simulink model "MultirotorSimulation"  (R2015b)
settings: Solver=VariableStepAuto  StartTime=0.0  StopTime=100  RelTol=1e-3
undefined symbols (not defined in the file): Initial, Motor, Uav
libraries: QuaternionLibrary x7
settings Model: Creator=jban039  LastModifiedBy=jeremie
settings ModelReferenceCC: ModelReferenceMinAlgLoopOccurrences=on

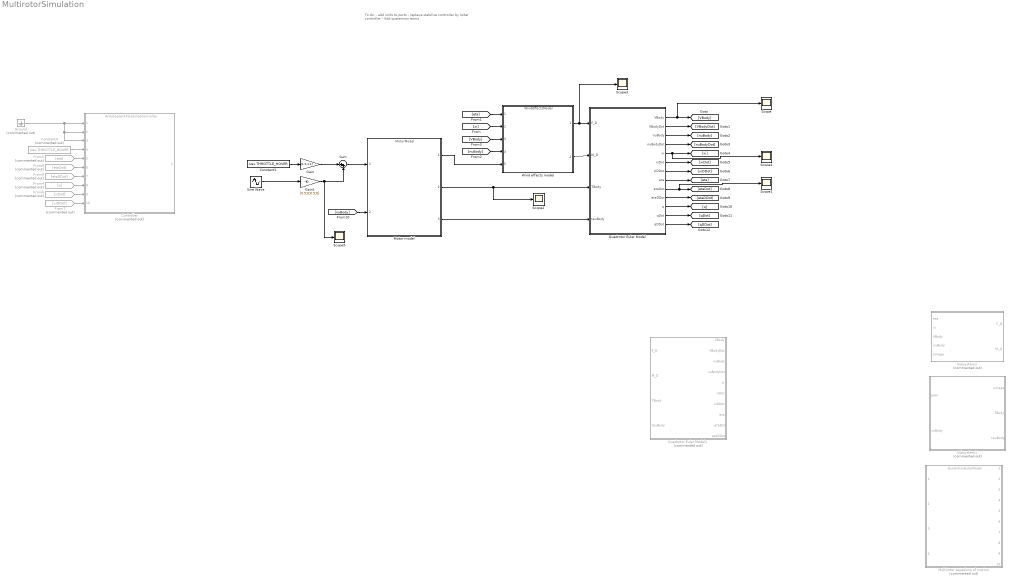
== system MultirotorSimulation ==
  note: To do:
      |
      | - add units  to ports
      | - replace stabilize controller by loiter controller
      | - Add quaternion eoms
  Constant1 : Constant  Value=Uav.THROTTLE_HOVER
  Constant4 : Constant  Commented=on  Value=Uav.THROTTLE_HOVER
  Controller : ModelReference  Commented=on  ModelNameDialog=ArduCopter33StabilizeController  SimulationMode=Normal  ModelReferenceVersion=1.9  CopyOfModelName=ArduCopter33StabilizeController
  From4 : From  Commented=on  GotoTag=xi
  From5 : From  Commented=on  GotoTag=eta
  From6 : From  Commented=on  GotoTag=xiDot
  From7 : From  Commented=on  GotoTag=xiDDot
  From8 : From  Commented=on  GotoTag=etaDot
  From9 : From  Commented=on  GotoTag=etaDDot
  Gain : Gain  Gain=[1;1;1;1]
  Gain1 : Gain  Gain=[0.5;0;0.5;0]
  Ground : Ground  Commented=on
  Motor model : ModelReference  ModelNameDialog=MotorModel  SimulationMode=Normal  ModelReferenceVersion=1.107  CopyOfModelName=MotorModel
  Multirotor equations of motion : ModelReference  Commented=on  ModelNameDialog=QuadrotorEulerModel  SimulationMode=Normal  ModelReferenceVersion=1.104  CopyOfModelName=QuadrotorEulerModel
  Quadrotor Euler Model : Subsystem
  Quadrotor Euler Model1 : Subsystem  Commented=on
  Scope{,1..5} (6 alike) : Scope
  Sine Wave : Sin  Amplitude=30  SampleTime=0
  Subsystem1 : Subsystem  Commented=on
  Subsystem2 : Subsystem  Commented=on
  Sum : Sum  Inputs=|++
  Wind effects model : ModelReference  ModelNameDialog=WindEffectsModel  SimulationMode=Normal  ModelReferenceVersion=1.49  CopyOfModelName=WindEffectsModel
  wires:
  Motor model/1 -> Wind effects model/5
  Motor model/2 -> Scope2/1, Quadrotor Euler Model/3(TBody)
  Motor model/3 -> Quadrotor Euler Model/4(tauBody)
  Wind effects model/2 -> Quadrotor Euler Model/2(M_D)
  Quadrotor Euler Model/1(VBody) -> Scope/1, [VBody]
  Quadrotor Euler Model/2(VBodyDot) -> [VBodyDot]
  Quadrotor Euler Model/3(nuBody) -> [nuBody]
  Quadrotor Euler Model/4(nuBodyDot) -> [nuBodyDot]
  Quadrotor Euler Model/5(xi) -> Scope4/1, [xi]
  Quadrotor Euler Model/6(xiDot) -> [xiDot]
  Quadrotor Euler Model/7(xiDDot) -> [xiDDot]
  Quadrotor Euler Model/8(eta) -> [eta]
  Quadrotor Euler Model/9(etaDot) -> Scope1/1, [etaDot]
  Quadrotor Euler Model/10(etaDDot) -> [etaDDot]
  [eta] -> Wind effects model/1
  [xi] -> Wind effects model/2
  [nuBody] -> Wind effects model/4
  [VBody] -> Wind effects model/3
  From5/1 -> Controller/5
  From4/1 -> Controller/8
  From6/1 -> Controller/9
  From7/1 -> Controller/10
  From8/1 -> Controller/6
  From9/1 -> Controller/7
  Ground/1 -> Controller/3, Controller/2, Controller/1
  Constant4/1 -> Controller/4
  [nuBody] -> Motor model/2
  Gain/1 -> Sum/1
  Constant1/1 -> Gain/1
  Sum/1 -> Motor model/1
  Gain1/1 -> Scope5/1, Sum/2
  Sine Wave/1 -> Gain1/1
  Quadrotor Euler Model/11(q) -> [q]
  Quadrotor Euler Model/12(qDot) -> [qDot]
  Quadrotor Euler Model/13(qDDot) -> [qDDot]
  Wind effects model/1 -> Scope3/1, Quadrotor Euler Model/1(F_D)

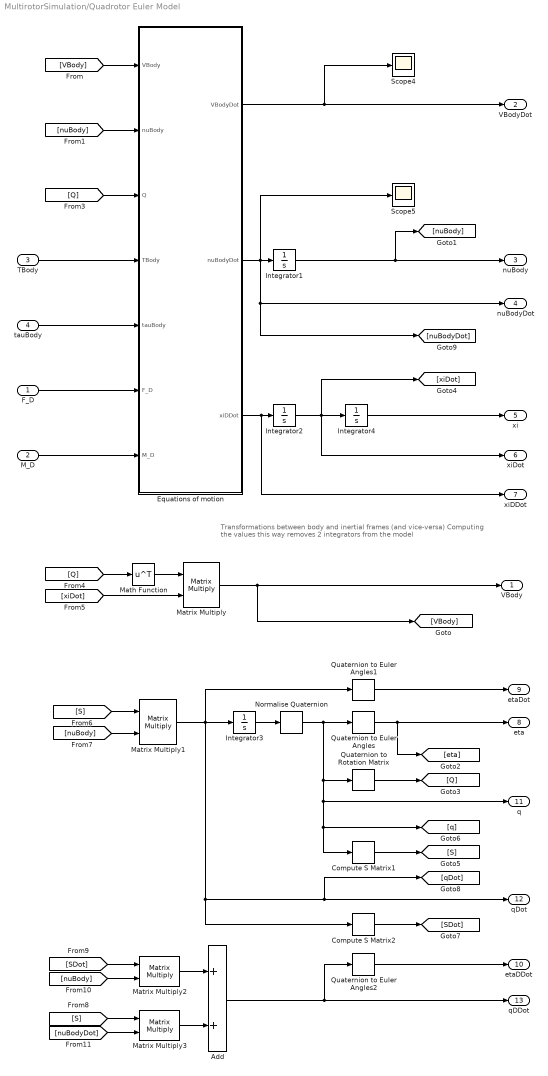
== system MultirotorSimulation/Quadrotor Euler Model ==
  note: Transformations between body and inertial frames (and vice-versa)
      | Computing the values this way removes 2 integrators from the model
  F_D : Inport
  M_D : Inport  Port=2
  TBody : Inport  Port=3
  tauBody : Inport  Port=4
  Add : Sum
  Compute S Matrix1 : QuaternionLibrary/Compute S Matrix
  Compute S Matrix2 : QuaternionLibrary/Compute S Matrix
  Equations of motion : MATLAB Function  TreatAsAtomicUnit=on
  Integrator1 : Integrator  InitialCondition=Initial.NU_BODY
  Integrator2 : Integrator  InitialCondition=Initial.XI_DOT
  Integrator3 : Integrator  InitialCondition=[0;0;0;1]
  Integrator4 : Integrator  InitialCondition=Initial.XI
  Math Function : Math  Operator=transpose  SaturateOnIntegerOverflow=on
  Matrix Multiply{,1..3} (4 alike) : Product  Multiplication=Matrix(*)
  Normalise Quaternion : QuaternionLibrary/Normalise Quaternion
  Quaternion to Euler Angles : QuaternionLibrary/Quaternion to Euler Angles
  Quaternion to Euler Angles1 : QuaternionLibrary/Quaternion to Euler Angles
  Quaternion to Euler Angles2 : QuaternionLibrary/Quaternion to Euler Angles
  Quaternion to Rotation Matrix : QuaternionLibrary/Quaternion to Rotation Matrix
  Scope4 : Scope
  Scope5 : Scope
  VBody : Outport
  VBodyDot : Outport  Port=2
  nuBody : Outport  Port=3
  nuBodyDot : Outport  Port=4
  xi : Outport  Port=5
  xiDot : Outport  Port=6
  xiDDot : Outport  Port=7
  eta : Outport  Port=8
  etaDot : Outport  Port=9
  etaDDot : Outport  Port=10
  q : Outport  Port=11
  qDot : Outport  Port=12
  qDDot : Outport  Port=13
  wires:
  Equations of motion/1(VBodyDot) -> VBodyDot/1, Scope4/1
  Integrator2/1 -> Integrator4/1, [xiDot], xiDot/1
  Integrator4/1 -> xi/1
  [nuBody] -> Equations of motion/2(nuBody)
  [VBody] -> Equations of motion/1(VBody)
  tauBody/1 -> Equations of motion/5(tauBody)
  TBody/1 -> Equations of motion/4(TBody)
  Equations of motion/3(xiDDot) -> Integrator2/1, xiDDot/1
  F_D/1 -> Equations of motion/6(F_D)
  Matrix Multiply/1 -> VBody/1, [VBody]
  M_D/1 -> Equations of motion/7(M_D)
  Integrator1/1 -> [nuBody], nuBody/1
  Equations of motion/2(nuBodyDot) -> Integrator1/1, nuBodyDot/1, [nuBodyDot], Scope5/1
  Integrator3/1 -> Normalise Quaternion/1
  Quaternion to Euler Angles/1 -> eta/1, [eta]
  Quaternion to Euler Angles1/1 -> etaDot/1
  Quaternion to Rotation Matrix/1 -> [Q]
  [Q] -> Equations of motion/3(Q)
  [Q] -> Math Function/1
  [xiDot] -> Matrix Multiply/2
  Math Function/1 -> Matrix Multiply/1
  [S] -> Matrix Multiply1/1
  [nuBody] -> Matrix Multiply1/2
  Compute S Matrix2/1 -> [SDot]
  [S] -> Matrix Multiply3/1
  Matrix Multiply1/1 -> Quaternion to Euler Angles1/1, qDot/1, [qDot], Compute S Matrix2/1, Integrator3/1
  [SDot] -> Matrix Multiply2/1
  [nuBody] -> Matrix Multiply2/2
  [nuBodyDot] -> Matrix Multiply3/2
  Matrix Multiply2/1 -> Add/1
  Matrix Multiply3/1 -> Add/2
  Add/1 -> Quaternion to Euler Angles2/1, qDDot/1
  Normalise Quaternion/1 -> Quaternion to Euler Angles/1, q/1, Compute S Matrix1/1, [q], Quaternion to Rotation Matrix/1
  Compute S Matrix1/1 -> [S]
  Quaternion to Euler Angles2/1 -> etaDDot/1

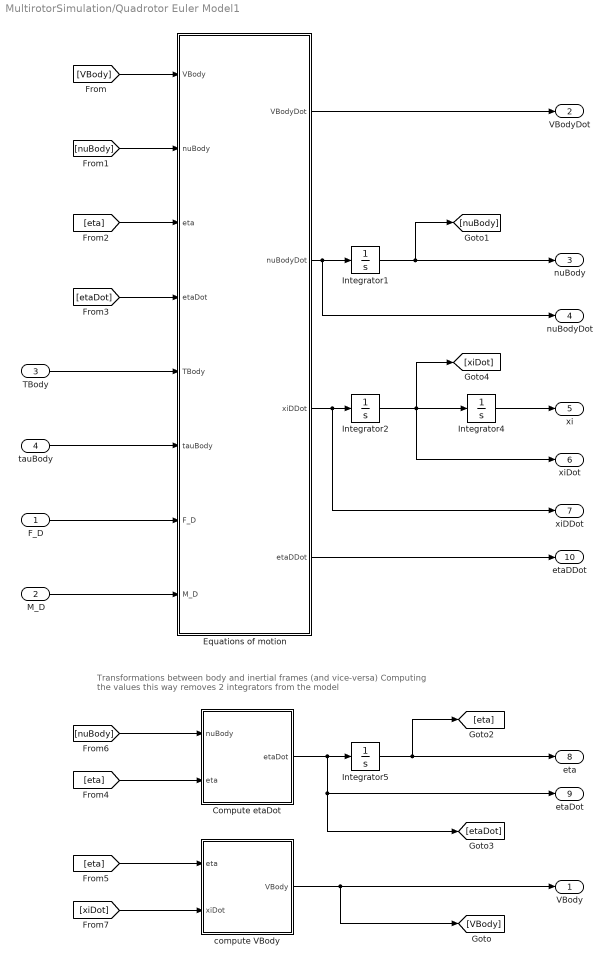
== system MultirotorSimulation/Quadrotor Euler Model1 ==
  note: Transformations between body and inertial frames (and vice-versa)
      | Computing the values this way removes 2 integrators from the model
  F_D : Inport
  M_D : Inport  Port=2
  TBody : Inport  Port=3
  tauBody : Inport  Port=4
  Compute etaDot : MATLAB Function  TreatAsAtomicUnit=on
  Equations of motion : MATLAB Function  TreatAsAtomicUnit=on
  Integrator1 : Integrator  InitialCondition=Initial.NU_BODY
  Integrator2 : Integrator  InitialCondition=Initial.XI_DOT
  Integrator4 : Integrator  InitialCondition=Initial.XI
  Integrator5 : Integrator  InitialCondition=Initial.ETA
  compute VBody : MATLAB Function  TreatAsAtomicUnit=on
  VBody : Outport
  VBodyDot : Outport  Port=2
  nuBody : Outport  Port=3
  nuBodyDot : Outport  Port=4
  xi : Outport  Port=5
  xiDot : Outport  Port=6
  xiDDot : Outport  Port=7
  eta : Outport  Port=8
  etaDot : Outport  Port=9
  etaDDot : Outport  Port=10
  wires:
  [xiDot] -> compute VBody/2(xiDot)
  [nuBody] -> Compute etaDot/1(nuBody)
  Equations of motion/2(nuBodyDot) -> Integrator1/1, nuBodyDot/1
  Integrator1/1 -> nuBody/1, [nuBody]
  M_D/1 -> Equations of motion/8(M_D)
  [eta] -> compute VBody/1(eta)
  compute VBody/1(VBody) -> VBody/1, [VBody]
  [eta] -> Compute etaDot/2(eta)
  Compute etaDot/1(etaDot) -> etaDot/1, [etaDot], Integrator5/1
  F_D/1 -> Equations of motion/7(F_D)
  Equations of motion/4(etaDDot) -> etaDDot/1
  Equations of motion/3(xiDDot) -> xiDDot/1, Integrator2/1
  TBody/1 -> Equations of motion/5(TBody)
  tauBody/1 -> Equations of motion/6(tauBody)
  [etaDot] -> Equations of motion/4(etaDot)
  [eta] -> Equations of motion/3(eta)
  Integrator5/1 -> [eta], eta/1
  [VBody] -> Equations of motion/1(VBody)
  [nuBody] -> Equations of motion/2(nuBody)
  Integrator4/1 -> xi/1
  Integrator2/1 -> xiDot/1, Integrator4/1, [xiDot]
  Equations of motion/1(VBodyDot) -> VBodyDot/1

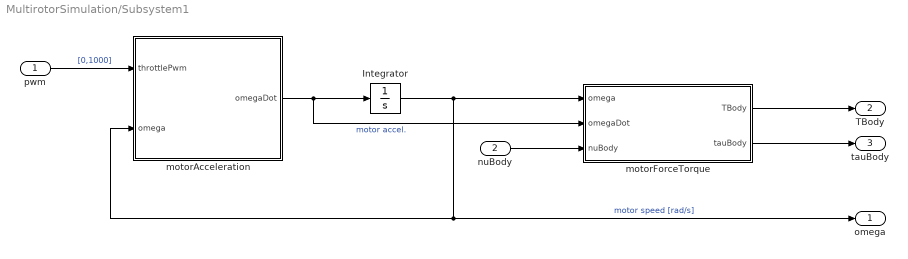
== system MultirotorSimulation/Subsystem1 ==
  pwm : Inport
  nuBody : Inport  Port=2
  Integrator : Integrator  InitialCondition=Initial.OMEGA
  motorAcceleration : MATLAB Function  TreatAsAtomicUnit=on
  motorForceTorque : MATLAB Function  TreatAsAtomicUnit=on
  omega : Outport
  TBody : Outport  Port=2
  tauBody : Outport  Port=3
  wires:
  motorAcceleration/1(omegaDot) -> motorForceTorque/2(omegaDot), Integrator/1  "motor accel."
  motorForceTorque/2(tauBody) -> tauBody/1
  motorForceTorque/1(TBody) -> TBody/1
  Integrator/1 -> motorForceTorque/1(omega), motorAcceleration/2(omega), omega/1  "motor speed [rad/s]"
  pwm/1 -> motorAcceleration/1(throttlePwm)  "[0,1000]"
  nuBody/1 -> motorForceTorque/3(nuBody)

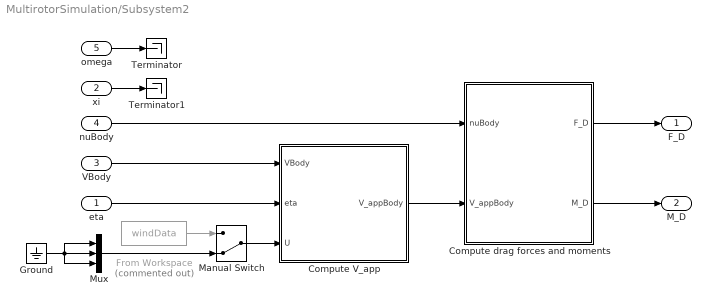
== system MultirotorSimulation/Subsystem2 ==
  eta : Inport  PortDimensions=3
  xi : Inport  Port=2  PortDimensions=3
  VBody : Inport  Port=3  PortDimensions=3
  nuBody : Inport  Port=4  PortDimensions=3
  omega : Inport  Port=5  PortDimensions=Uav.N_ROTORS
  Compute V_app : MATLAB Function  TreatAsAtomicUnit=on
  Compute drag forces and moments : MATLAB Function  TreatAsAtomicUnit=on
  From Workspace : FromWorkspace  Commented=on  VariableName=windData  SampleTime=0
  Ground : Ground
  Manual Switch : ManualSwitch  CurrentSetting=0
  Mux : Mux  Inputs=3
  Terminator : Terminator
  Terminator1 : Terminator
  F_D : Outport
  M_D : Outport  Port=2
  wires:
  Compute drag forces and moments/1(F_D) -> F_D/1
  Compute drag forces and moments/2(M_D) -> M_D/1
  Compute V_app/1(V_appBody) -> Compute drag forces and moments/2(V_appBody)
  omega/1 -> Terminator/1
  Manual Switch/1 -> Compute V_app/3(U)
  xi/1 -> Terminator1/1
  Ground/1 -> Mux/1, Mux/3, Mux/2
  From Workspace/1 -> Manual Switch/1
  Mux/1 -> Manual Switch/2
  nuBody/1 -> Compute drag forces and moments/1(nuBody)
  VBody/1 -> Compute V_app/1(VBody)
  eta/1 -> Compute V_app/2(eta)

== matlab function MultirotorSimulation/Quadrotor Euler Model/Equations of motion ==
  data: VBody input; VBodyDot output; nuBody input; Q input; TBody input size=3; tauBody input size=3; F_D input size=3; M_D input size=3; nuBodyDot output; Uav parameter; xiDDot output
function [VBodyDot, nuBodyDot, xiDDot] = QuadrotorEulerModel(...
    VBody, nuBody, Q, TBody, tauBody, F_D, M_D, Uav)
%#codegen

%% Rotation matrices

%% Moments and Forces
% Body frame accelerations
VBodyDot  = (1/Uav.M) * (Q'*Uav.G + TBody - cross(nuBody, Uav.M*VBody) - F_D);
nuBodyDot = Uav.I \ (tauBody - cross(nuBody, Uav.I*nuBody) - M_D);

% Inertial frame accelerations
xiDDot = (1/Uav.M)*(Uav.G + Q*TBody - Q*F_D);
% etaDDot = WInvertDot*nuBody + WInvert*nuBodyDot;

% Check centripetal force in inertial frame
% F_C = R*cross(nuBody,m*VBody);
end

== matlab function MultirotorSimulation/Subsystem2/Compute V_app ==
  data: VBody input; eta input; V_appBody output; U input size=3
function V_appBody = computeV_appBody(VBody, eta, U)
%#codegen

sPhi   = sin(eta(1));
sTheta = sin(eta(2));
sPsi   = sin(eta(3));
cPhi   = cos(eta(1));
cTheta = cos(eta(2));
cPsi   = cos(eta(3));

R = [cPsi*cTheta, cPsi*sTheta*sPhi-sPsi*cPhi, cPsi*sTheta*cPhi+sPsi*sPhi;
     sPsi*cTheta, sPsi*sTheta*sPhi+cPsi*cPhi, sPsi*sTheta*cPhi-cPsi*sPhi;
     -sTheta,     cTheta*sPhi,                cTheta*cPhi+sPsi*sPhi];

% Rotation matrix from Wind frame to Inertial frame 
R_U = [1, 0,  0;
       0, 1,  0;
       0, 0, -1];

V_appBody = VBody + R'*R_U*U;

== matlab function MultirotorSimulation/Subsystem2/Compute drag forces and moments ==
  data: nuBody input; V_appBody input; F_D output; M_D output; Uav parameter
function [F_D, M_D] = computeDrag(nuBody, V_appBody, Uav)
%#codegen

% Calculate drag force
F_D = 0.5 * Uav.RHO_AIR * Uav.C_D * (abs(V_appBody) .* V_appBody);

% Drag moment, applied to independent axes
M_D = 0.5 * Uav.RHO_AIR * Uav.C_DM * (abs(nuBody) .* nuBody);

== matlab function MultirotorSimulation/Quadrotor Euler Model1/Compute etaDot ==
  data: nuBody input; eta input; etaDot output
function etaDot = computeEtaDot(nuBody, eta)
%#codegen

sPhi = sin(eta(1));
cPhi = cos(eta(1));
cTheta = cos(eta(2));
tTheta = tan(eta(2));
      
WInverse = [1, sPhi*tTheta,  cPhi*tTheta;
            0, cPhi,        -sPhi;
            0, sPhi/cTheta,  cPhi/cTheta];

etaDot = WInverse*nuBody;

== matlab function MultirotorSimulation/Quadrotor Euler Model1/Equations of motion ==
  data: VBody input; VBodyDot output; nuBody input; eta input; etaDot input; TBody input size=3; tauBody input size=3; F_D input size=3; M_D input size=3; nuBodyDot output; Uav parameter; xiDDot output; etaDDot output
function [VBodyDot, nuBodyDot, xiDDot, etaDDot] = QuadrotorEulerModel(...
    VBody, nuBody, eta, etaDot, TBody, tauBody, F_D, M_D, Uav)
%#codegen

%% Rotation matrices
% Precompute sines and cosines
sPhi   = sin(eta(1));
sTheta = sin(eta(2));
sPsi   = sin(eta(3));
cPhi   = cos(eta(1));
cTheta = cos(eta(2));
cPsi   = cos(eta(3));
tTheta = tan(eta(2));

phiDot   = etaDot(1);
thetaDot = etaDot(2);

% Body frame to inertial frame
R = [cPsi*cTheta, cPsi*sTheta*sPhi-sPsi*cPhi, cPsi*sTheta*cPhi+sPsi*sPhi;
     sPsi*cTheta, sPsi*sTheta*sPhi+cPsi*cPhi, sPsi*sTheta*cPhi-cPsi*sPhi;
     -sTheta,     cTheta*sPhi,                cTheta*cPhi+sPsi*sPhi];

WInvertDot = [...
    0,  phiDot*cPhi*tTheta+thetaDot*sPhi/cTheta^2,    -phiDot*sPhi*cTheta+thetaDot*cPhi/cTheta^2;
    0, -phiDot*sPhi,                                  -phiDot*cPhi;
	0,  phiDot*cPhi/cTheta+phiDot*sPhi*tTheta/cTheta, -phiDot*sPhi/cTheta+thetaDot*cPhi*tTheta/cTheta];

WInvert = [1, sPhi*tTheta,  cPhi*tTheta;
           0, cPhi,        -sPhi;
           0, sPhi/cTheta,  cPhi/cTheta];

%% Moments and Forces
% Body frame accelerations
VBodyDot  = (1/Uav.M) * (R'*Uav.G + TBody - cross(nuBody, Uav.M*VBody) - F_D);
nuBodyDot = Uav.I \ (tauBody - cross(nuBody, Uav.I*nuBody) - M_D);

% Inertial frame accelerations
xiDDot = (1/Uav.M)*(Uav.G + R*TBody - R*F_D);
etaDDot = WInvertDot*nuBody + WInvert*nuBodyDot;

% Check centripetal force in inertial frame
% F_C = R*cross(nuBody,m*VBody);
end

function S = computeS(q)
    S = 0.5 .* [-q(1), -q(2), -q(3);
                 q(0), -q(3),  q(2);
                 q(3),  q(0), -q(1);
                -q(2),  q(1),  q(0)];
end

== matlab function MultirotorSimulation/Quadrotor Euler Model1/compute VBody ==
  data: eta input; VBody output; xiDot input
function VBody = computeVBody(eta, xiDot)
%#codegen

sphi = sin(eta(1));
sTheta = sin(eta(2));
sPsi = sin(eta(3));
cPhi = cos(eta(1));
cTheta = cos(eta(2));
cPsi = cos(eta(3));

R = [ cPsi*cTheta, cPsi*sTheta*sphi-sPsi*cPhi, cPsi*sTheta*cPhi+sPsi*sphi;
	  sPsi*cTheta, sPsi*sTheta*sphi+cPsi*cPhi, sPsi*sTheta*cPhi-cPsi*sphi;
     -sTheta,      cTheta*sphi,                cTheta*cPhi+sPsi*sphi];

VBody = R'*xiDot;

== matlab function MultirotorSimulation/Subsystem1/motorForceTorque ==
  data: omega input; TBody output; omegaDot input; nuBody input size=3; Motor parameter; Uav parameter; tauBody output
function [TBody, tauBody] = motorForceTorque(...
    omega, omegaDot, nuBody, Motor, Uav)
%#codegen

% Make assertions to avoid code generation errors
assert(Uav.N_ROTORS < 16);

%% Thrust and differential torque

% Concatenated motor force/torque vectors in respective motor frame
% eg. TMotor = [TMotor1, TMotor2, ..., TMotorN]
% where: - N is the number of rotors
%        - TMotorx (x ∈ [1,2,...,N]) is the thrust generated by motor x in
%          its own frame of reference
TMotorIndividual = [ zeros(2, Uav.N_ROTORS);
           Motor.K * (omega'.^2) ];
tauMotorIndividual = [ zeros(2, Uav.N_ROTORS);
             Uav.ROTOR_DIRECTION .* ...
                 ( Motor.B*(omega'.^2) + Motor.I_R(3,3)*omegaDot' ) ];

% Initialise matrices to store motor force/torque vectors in body frame
TBodyIndividual   = zeros(3, Uav.N_ROTORS);
tauBodyIndividual = zeros(3, Uav.N_ROTORS);

% Calculate forces and moments from each motor in the body frame
for i = 1:Uav.N_ROTORS
    l = Uav.L(i);
    beta = Uav.BETA(i);
    
 	RMotorToBody = [ 0,            0,            l*sin(beta);
                     0,            0,           -l*cos(beta);
                    -l*sin(beta),  l*cos(beta),  0 ];

	% Motor force/torque vectors in body frame - need rotation matrix for
	% canted rotors(!)
	TBodyIndividual(:,i) = TMotorIndividual(:,i);
	tauBodyIndividual(:,i) = tauMotorIndividual(:,i) + ...
        RMotorToBody * TMotorIndividual(:,i);
end

%% Gyroscopic moments

% Concatenated gyroscopic moments for each rotor
M_GBodyIndividual = zeros(3, Uav.N_ROTORS);

% Concatenated motor speeds in their respective frames
omegaMotor = [ zeros(2, Uav.N_ROTORS);
               Uav.ROTOR_DIRECTION .* omega' ];
           
% Angular momentum in motor frame
H_MMotorSeparate = Motor.I_R * omegaMotor;

% Gyroscopic moment vectors in body frame
for i = 1:Uav.N_ROTORS
	M_GBodyIndividual(:,i) = cross(nuBody, H_MMotorSeparate(:,i));
end

M_GBody = sum(M_GBodyIndividual, 2);

%% Total torque and moment

% Total force/torque in body frame
TBody = sum(TBodyIndividual, 2);
tauBody = sum(tauBodyIndividual, 2) + M_GBody;

end

== matlab function MultirotorSimulation/Subsystem1/motorAcceleration ==
  data: throttlePwm input; omegaDot output double size=4; omega input; Motor parameter; Uav parameter
function omegaDot = motorAcceleration(throttlePwm, omega, Motor, Uav)
%#codegen

voltage = throttlePwm * Uav.NOMINAL_BATTERY_VOLTAGE / 1000;

% Motor current ignoring inductance
current = (voltage - Motor.K_E*omega) / Motor.R;

netTorque = (Motor.K_T * current) - (Motor.B * omega.^2);

% Motor angular acceleration
omegaDot = netTorque / Motor.I_R(3,3);
